simulink model "untitled"  (R2016a)
settings: Solver=VariableStepAuto  StartTime=0.0  StopTime=10.0  RelTol=1e-3
settings Model: Creator=Użytkownik  LastModifiedBy=Użytkownik

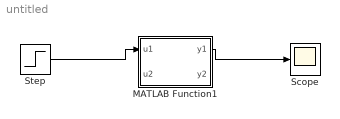
== system untitled ==
  MATLAB Function1 : MATLAB Function  TreatAsAtomicUnit=on
  Scope : Scope
  Step : Step  SampleTime=0
  wires:
  Step/1 -> MATLAB Function1/1(u1)
  MATLAB Function1/1(y1) -> Scope/1

== matlab function untitled/MATLAB Function1 ==
  data: u1 input; y1 output; y2 output; u2 input
function [y1, y2] = fcn(u1, u2)

a = [(1/10)*u, (1/5)*u, u];
%#codegen

y = a;
